simulink subsystem "Perturbation_ESC"  (R2024b)
settings: Solver=VariableStepAuto  StartTime=0.0  StopTime=10.0  RelTol=1e-3
undefined symbols (not defined in the file or in its folder): a, C, esc_ic, g, M, magnitude, omega, phi, x_c, x_l
settings Model: Creator=Henrique Mesquita  LastModifiedBy=LCA
settings DebuggingCC: UnconnectedInputMsg=warning  UnconnectedOutputMsg=warning  UnconnectedLineMsg=warning
settings ModelReferenceCC: EnableRefExpFcnMdlSchedulingChecks=on
settings RTWCC: GPUComputeCapability=3.5  DLArmComputeVersion=19.05

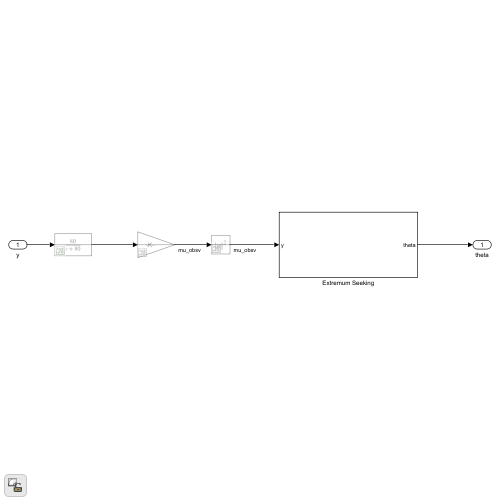
[thumbnail: Simulink's stored preview of the top-level diagram]
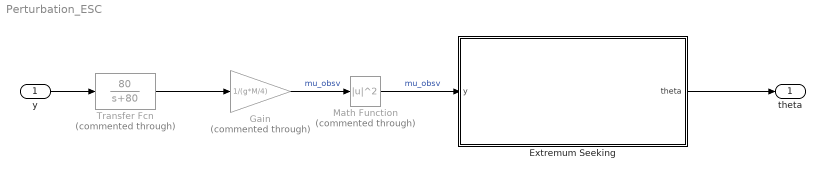
== system Perturbation_ESC ==
  y : Inport
  Extremum Seeking : Subsystem
  Gain : Gain  Commented=through  Gain=1/(g*M/4)
  Math Function : Math  Commented=through  Operator=magnitude^2
  Transfer Fcn : TransferFcn  Commented=through  Numerator=[80]  Denominator=[1 80]
  theta : Outport
  wires:
  Transfer Fcn/1 -> Gain/1
  Gain/1 -> Math Function/1  "mu_obsv"
  Extremum Seeking/1(theta) -> theta/1
  Math Function/1 -> Extremum Seeking/1(y)  "mu_obsv"
  y/1 -> Transfer Fcn/1

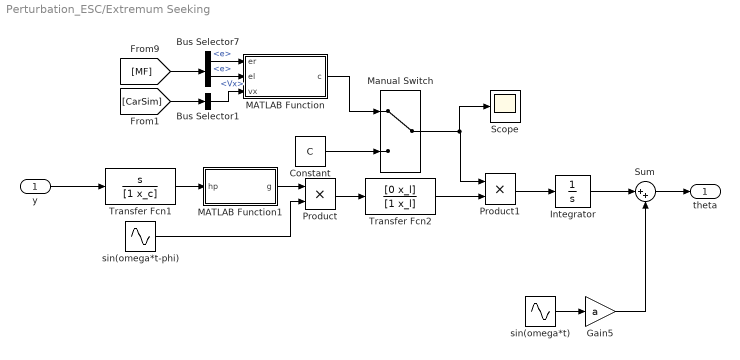
== system Perturbation_ESC/Extremum Seeking ==
  y : Inport
  Bus Selector1 : BusSelector  OutputSignals=Vx
  Bus Selector7 : BusSelector  OutputSignals=info (signal 1).e,info (signal 2).e
  Constant : Constant  Value=C
  Gain5 : Gain  Gain=a
  Integrator : Integrator  InitialCondition=esc_ic  LimitOutput=on  UpperSaturationLimit=0.2  LowerSaturationLimit=0.01
  MATLAB Function : MATLAB Function  TreatAsAtomicUnit=on
  MATLAB Function1 : MATLAB Function  TreatAsAtomicUnit=on
  Manual Switch : ManualSwitch
  Product : Product
  Product1 : Product
  Scope : Scope
  Sum : Sum  Inputs=|++
  Transfer Fcn1 : TransferFcn  Numerator=[1 0]  Denominator=[1 x_c]
  Transfer Fcn2 : TransferFcn  Numerator=[0 x_l]  Denominator=[1 x_l]
  sin(omega*t) : Sin  Frequency=omega  SampleTime=0
  sin(omega*t-phi) : Sin  Frequency=omega  Phase=phi  SampleTime=0
  theta : Outport
  wires:
  MATLAB Function1/1(g) -> Product/1
  Bus Selector1/1 -> MATLAB Function/3(vx)  "<Vx>"
  [CarSim] -> Bus Selector1/1
  Transfer Fcn1/1 -> MATLAB Function1/1(hp)
  Manual Switch/1 -> Product1/1, Scope/1
  Constant/1 -> Manual Switch/2
  MATLAB Function/1(c) -> Manual Switch/1
  Bus Selector7/2 -> MATLAB Function/2(el)  "<e>"
  Bus Selector7/1 -> MATLAB Function/1(er)  "<e>"
  [MF] -> Bus Selector7/1
  Integrator/1 -> Sum/1
  Product1/1 -> Integrator/1
  sin(omega*t-phi)/1 -> Product/2
  y/1 -> Transfer Fcn1/1
  Transfer Fcn2/1 -> Product1/2
  Product/1 -> Transfer Fcn2/1
  Sum/1 -> theta/1
  Gain5/1 -> Sum/2
  sin(omega*t)/1 -> Gain5/1

== matlab function Perturbation_ESC/Extremum Seeking/MATLAB Function ==
  data: er input; c output; el input; C parameter; vx input
function c = fcn(er, el, C, vx)

VMAX = 120;
VMIN = 3;

persistent de_ant;
persistent e_ant;
if(isempty(de_ant)||isempty(e_ant))
    de_ant = 0;
    e_ant = 0;
end

e = (er+el)/2;

% if(e^2<1e-4)
%     c = C;
% else
%     c = C*(exp(-(e^2)/0.0001));
% end
% c = C*(exp(-(e^2)/0.01));
% c=C;

if(vx>VMAX || vx<0.1)
    c=0;
else
%     c = min([C (VMAX-vx)/(VMAX-VMIN)*C]);
%     c = min([C exp(-(vx-VMIN)/(VMAX/5))*C]);
%     if c < C/30
%         c = C/30;
%     end
    c=C;
    c = c*(exp(-(e^2)/0.0002));
end
% de = 19.03*(e-e_ant)+0.9048*de_ant;
% 
% if(abs(e)>0.01 || abs(de)>0.05)
%     c=0;
% else
%     c = C;
% end

% if(j<=0)
%     y = 0;
% else
%     y = 200*j;
% end

== matlab function Perturbation_ESC/Extremum Seeking/MATLAB Function1 ==
  data: hp input; g output
function g = demAmp(hp)

% if(abs(hp)>0.05)
%     g = hp*(exp(-(abs(hp)-0.05)/0.01));
% else
%     g = hp;
% end

% g = hp*(exp(-hp^2/0.005));
g = hp;
